simulink library "UtilityLibrary"  (R2021a)
settings: Solver=VariableStepAuto  StartTime=0.0  StopTime=10.0  RelTol=1e-3
libraries: simulink x1, $bdroot x1
settings Model: Creator=phill  LastModifiedBy=phill

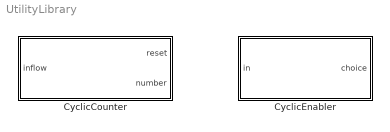
== system UtilityLibrary ==
  CyclicCounter : Subsystem  mask{resetThreshold=1}
      mask prompts: resetThreshold "reset threshold"
      mask Display:
      | disp('flow ctr \n\n');
      | disp(['resets at x = ', get_param(gcb,'resetThreshold')])
  CyclicEnabler : Subsystem  mask{resetThreshold=1}
      mask prompts: resetThreshold "reset threshold"
      mask Display:
      | disp('Cyc Enabler \n\n');
      | disp(['resets at x = ', get_param(gcb,'resetThreshold')])

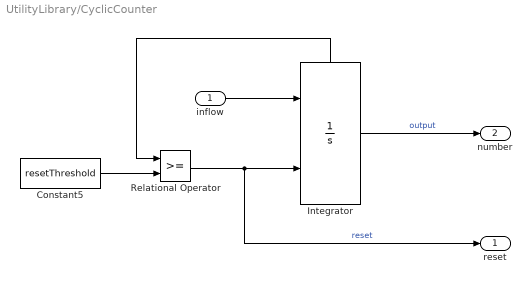
== system UtilityLibrary/CyclicCounter ==
  inflow : Inport
  Constant5 : Constant  Value=resetThreshold
  Integrator : Integrator  ExternalReset=rising  LimitOutput=on  UpperSaturationLimit=resetThreshold  LowerSaturationLimit=0  ShowStatePort=on
  Relational Operator : RelationalOperator  OutDataTypeStr=boolean  RndMeth=Simplest
  reset : Outport
  number : Outport  Port=2
  wires:
  Constant5/1 -> Relational Operator/2
  Integrator/1 -> number/1  "output"
  inflow/1 -> Integrator/1
  Relational Operator/1 -> Integrator/2, reset/1  "reset"
  Integrator/State -> Relational Operator/1

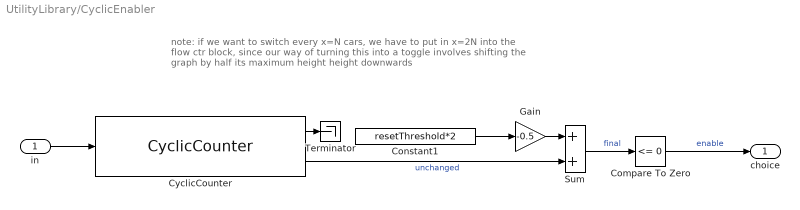
== system UtilityLibrary/CyclicEnabler ==
  note: note: if we want to switch every x=N cars, we have to put in x=2N
      | into the flow ctr block, since our way of turning this into a toggle involves
      | shifting the graph by half its maximum height height downwards
  in : Inport
  Compare To Zero : simulink/Logic and Bit Operations/Compare To Zero  relop=<=  OutDataTypeStr=boolean
  Constant1 : Constant  Value=resetThreshold*2
  CyclicCounter : $bdroot/CyclicCounter  resetThreshold=resetThreshold*2
  Gain : Gain  Gain=-0.5
  Sum : Sum
  Terminator : Terminator
  choice : Outport
  wires:
  CyclicCounter/1 -> Terminator/1
  CyclicCounter/2 -> Sum/2  "unchanged"
  Constant1/1 -> Gain/1
  Gain/1 -> Sum/1
  Sum/1 -> Compare To Zero/1  "final"
  in/1 -> CyclicCounter/1
  Compare To Zero/1 -> choice/1  "enable"
